simulink model "state_flow_chart"  (R2024a)
settings: Solver=VariableStepAuto  StartTime=0.0  StopTime=5  RelTol=1e-3
settings Model: Creator=mustafaenesozdel  LastModifiedBy=mustafaenesozdel

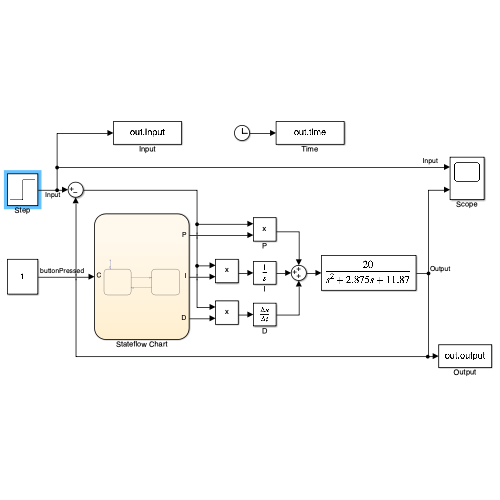
[thumbnail: Simulink's stored preview of the top-level diagram]
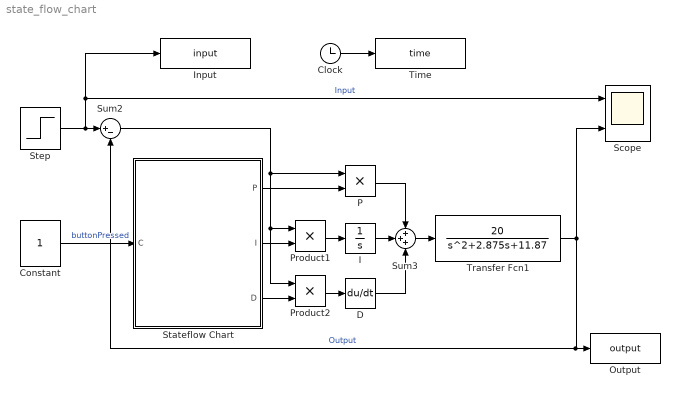
== system state_flow_chart ==
  Clock : Clock
  Constant : Constant
  D : Derivative
  I : Integrator
  Input : ToWorkspace  VariableName=input  SaveFormat=Timeseries  SampleTime=-1
  Output : ToWorkspace  VariableName=output  SaveFormat=Timeseries  SampleTime=-1
  P : Product
  Product1 : Product
  Product2 : Product
  Scope : Scope  NumInputPorts=2
  Stateflow Chart : Stateflow chart  TreatAsAtomicUnit=on
  Step : Step  Time=0.0001  SampleTime=0
  Sum2 : Sum  Inputs=|+-
  Sum3 : Sum  Inputs=+++
  Time : ToWorkspace  VariableName=time  SaveFormat=Timeseries  SampleTime=-1
  Transfer Fcn1 : TransferFcn  Numerator=[20]  Denominator=[1 2.875 11.87]
  wires:
  Sum2/1 -> Product2/1, Product1/1, P/1
  Constant/1 -> Stateflow Chart/1(C)  "buttonPressed"
  Clock/1 -> Time/1
  P/1 -> Sum3/1
  Sum3/1 -> Transfer Fcn1/1
  Step/1 -> Scope/1, Input/1, Sum2/1  "Input"
  I/1 -> Sum3/2
  D/1 -> Sum3/3
  Transfer Fcn1/1 -> Output/1, Sum2/2, Scope/2  "Output"
  Stateflow Chart/3(D) -> Product2/2
  Stateflow Chart/1(P) -> P/2
  Product1/1 -> I/1
  Stateflow Chart/2(I) -> Product1/2
  Product2/1 -> D/1

== stateflow chart state_flow_chart/Stateflow Chart ==
  state PID1
    during:
    P = P1;
    I = I1;
    D = D1;
  state PID2
    during:
    P = P2;
    I = I2;
    D = D2;
  (default) -> PID1
  PID1 -> PID2 : [C == 2]
  PID2 -> PID1 : [C == 1]
  data: C input; P output; I output; D output; D2 constant double =3; I1 constant double =0; I2 constant double =5; P2 constant double =50; D1 constant double =0; P1 constant double =1
